simulink model "ssb"  (R2019b)
settings: Solver=VariableStepAuto  StartTime=0.0  StopTime=10.0  RelTol=1e-3
undefined symbols (not defined in the file or in its folder): fdesignblkfcn, gcbh
libraries: commanapbnd3 x2, eeGeneralControl x1
settings Model: Creator=Win 10  LastModifiedBy=thuma

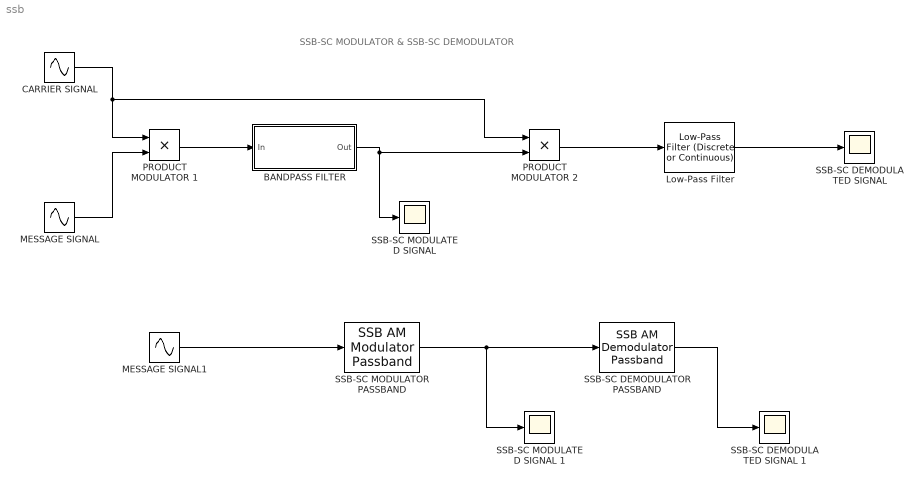
== system ssb ==
  note: SSB-SC MODULATOR & SSB-SC DEMODULATOR
  " Low-Pass Filter" : eeGeneralControl/Low-Pass Filter (Discrete or Continuous)  K=1  T=1  B=10  A=-10  Ts=0
      settings: SourceProductName=Simscape Electrical
  " SSB-SC DEMODULATOR PASSBAND" : commanapbnd3/SSB AM Demodulator Passband  Fc=25  Ph=0  method=Butterworth  n=8  cf=20  Rp=0.1  Rs=50
      settings: SourceProductName=Communications Toolbox  SourceProductBaseCode=CM
  " SSB-SC MODULATOR PASSBAND" : commanapbnd3/SSB AM Modulator Passband  Fc=25  Ph=0  Sd=Lower  Ho=100
      settings: SourceProductName=Communications Toolbox  SourceProductBaseCode=CM
  "BANDPASS FILTER " : Subsystem  DialogController=fdesignblkfcn  InitFcn=fdesignblkfcn(gcbh, {'InitFcn'});  mask(Bandpass Filter){}
      mask help: Design a bandpass filter
      settings: CopyFcn=fdesignblkfcn(gcbh, {'CopyFcn'});
      mask Help: helpview(mapfilelocation('dsp'), 'dspbandpassfilter');
      mask Display: disp('Bandpass');
  CARRIER SIGNAL : Sin  Frequency=2*pi*10  SampleTime=0.001
  MESSAGE SIGNAL : Sin  Frequency=2*pi*1  SampleTime=0.001
  MESSAGE SIGNAL1 : Sin  Frequency=2*pi*1  SampleTime=0.001
  PRODUCT MODULATOR 1 : Product
  PRODUCT MODULATOR 2 : Product
  SSB-SC DEMODULATED SIGNAL : Scope
  SSB-SC DEMODULATED SIGNAL 1 : Scope
  SSB-SC MODULATED SIGNAL : Scope
  SSB-SC MODULATED SIGNAL 1 : Scope
  wires:
  CARRIER SIGNAL/1 -> PRODUCT MODULATOR 2/1, PRODUCT MODULATOR 1/1
  MESSAGE SIGNAL/1 -> PRODUCT MODULATOR 1/2
  PRODUCT MODULATOR 1/1 -> "BANDPASS FILTER "/1(In)
  "BANDPASS FILTER "/1(Out) -> SSB-SC MODULATED SIGNAL/1, PRODUCT MODULATOR 2/2
  PRODUCT MODULATOR 2/1 -> " Low-Pass Filter"/1
  " Low-Pass Filter"/1 -> SSB-SC DEMODULATED SIGNAL/1
  MESSAGE SIGNAL1/1 -> " SSB-SC MODULATOR PASSBAND"/1
  " SSB-SC MODULATOR PASSBAND"/1 -> SSB-SC MODULATED SIGNAL 1/1, " SSB-SC DEMODULATOR PASSBAND"/1
  " SSB-SC DEMODULATOR PASSBAND"/1 -> SSB-SC DEMODULATED SIGNAL 1/1

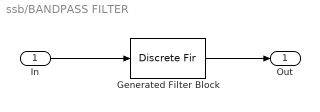
== system ssb/BANDPASS FILTER  ==
  In : Inport
  Generated Filter Block : DiscreteFir  Tag=BlockMethodSubSystem  Coefficients=[-0.153489825895129439 0.0570452397846297199 -0.0542597268841885569 0.0412204175720009697 -0.0182634618102462121 -0.0125219920876095472 0.0472298298247487841 -0.0813874699807817653 0.110517022709823581 -0.129700597986994987 0.136532324109984449 -0.129700597986994987 0.110517022709823581 -0.0813874699807817653 0.0472298298247487841 -0.0125219920876095472 -0.0182634618102462121 0.0412204175720009697 -0.0542597268841885569 0.0570452397846297199 -0.153489825895129439]  InputProcessing=Columns as channels (frame based)
  Out : Outport  VectorParamsAs1DForOutWhenUnconnected=off
  wires:
  In/1 -> Generated Filter Block/1
  Generated Filter Block/1 -> Out/1
